simulink model "canBusModel"  (R2024b)
settings: Solver=FixedStepDiscrete  StartTime=0.0  StopTime=2  FixedStep=0.00001  RelTol=1e-3
undefined symbols (not defined in the file): CanFDSpeed_bps, CanSpeed_bps, FixedStep_us
settings Model: Creator=junho  LastModifiedBy=hrkim
settings DebuggingCC: ModelReferenceSymbolNameMessage=none
settings HardwareCC: TargetBitPerLong=64  TargetBitPerPointer=64  TargetBitPerSizeT=64  TargetBitPerPtrDiffT=64  TargetLongLongMode=on  TargetIntDivRoundTo=Zero  TargetEndianess=LittleEndian  TargetWordSize=64  TargetHWDeviceType=MATLAB Host  ProdEqTarget=off
settings SFSimCC: SimUserSources=../src/canBus.c  DefaultCustomCodeDeterministicFunctions=ByFunction  CustomCodeDeterministicFunctions=fmu_can_init
settings SFSimCC: SimCustomHeaderCode=|
  | #include "../src/canBus.h";
  | #include "string.h";
settings RTWCC: Description=FMU2CS  SystemTargetFile=fmu2cs.tlc  TemplateMakefile=fmu2cs_default_tmf  RTWVerbose=off  RTWUseSimCustomCode=on  CustomSource=../src/canBus.c  GPUComputeCapability=3.5
settings RTWCC: CustomHeaderCode=|
  | #include "../src/canBus.h";
  | #include "string.h";
settings CodeAppCC: MaxIdLength=255
settings GRTTargetCC: MatFileLogging=off

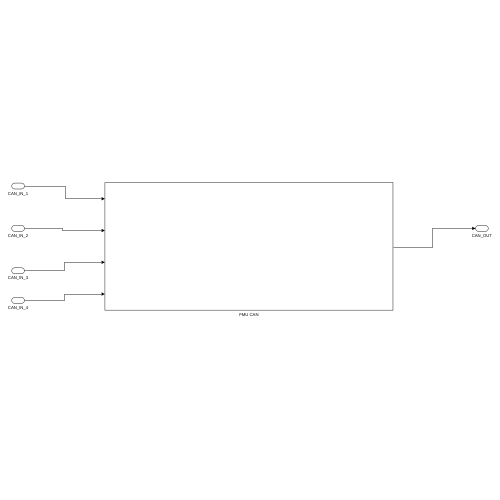
[thumbnail: Simulink's stored preview of the top-level diagram]
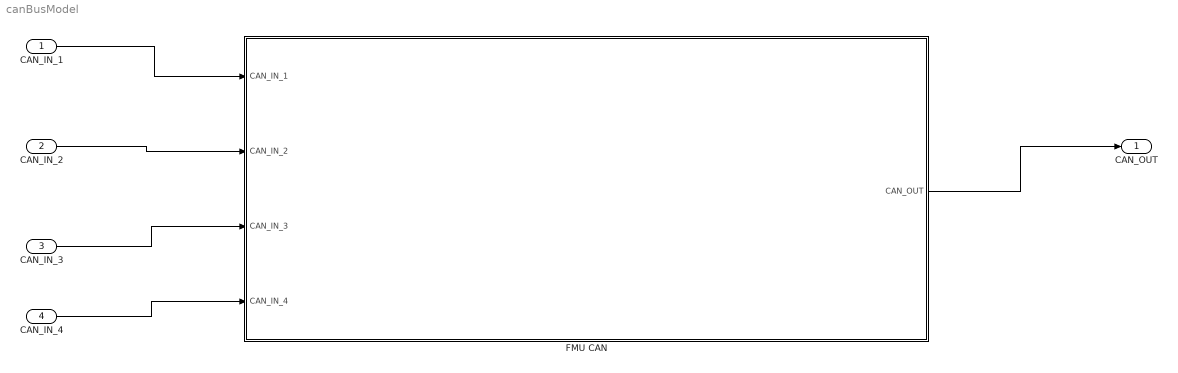
== system canBusModel ==
  CAN_IN_1 : Inport
  CAN_IN_2 : Inport  Port=2
  CAN_IN_3 : Inport  Port=3
  CAN_IN_4 : Inport  Port=4
  FMU CAN : Subsystem
  CAN_OUT : Outport
  wires:
  FMU CAN/1(CAN_OUT) -> CAN_OUT/1
  CAN_IN_1/1 -> FMU CAN/1(CAN_IN_1)
  CAN_IN_2/1 -> FMU CAN/2(CAN_IN_2)
  CAN_IN_3/1 -> FMU CAN/3(CAN_IN_3)
  CAN_IN_4/1 -> FMU CAN/4(CAN_IN_4)

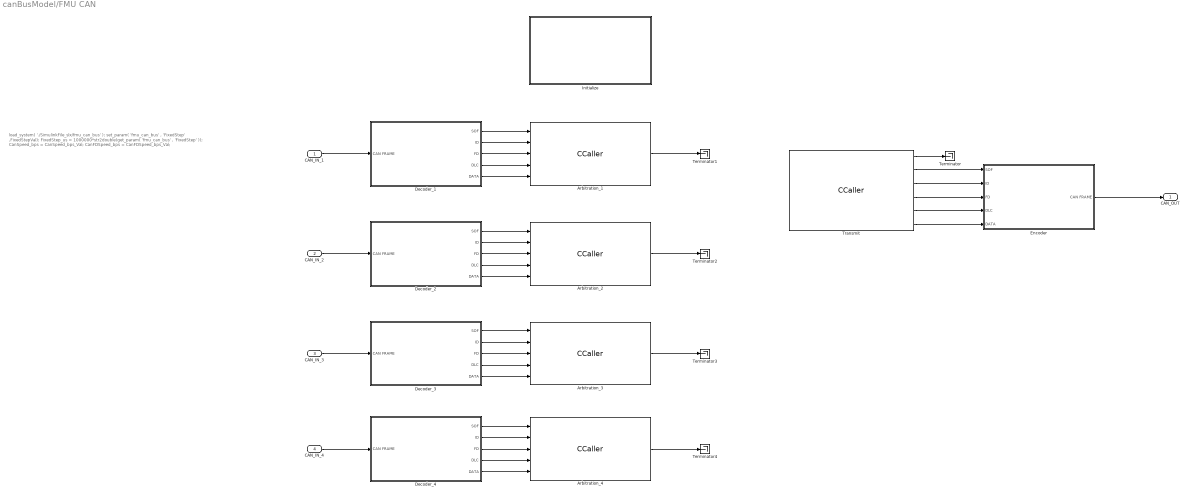
== system canBusModel/FMU CAN ==
  note: load_system( './SimulinkFile_slx/fmu_can_bus' );
      | set_param( 'fmu_can_bus' , 'FixedStep' ,FixedStepVal);
      | FixedStep_us = 1000000*str2double(get_param( 'fmu_can_bus' , 'FixedStep' ));
      | CanSpeed_bps = CanSpeed_bps_Val;
      | CanFDSpeed_bps = CanFDSpeed_bps_Val;
  CAN_IN_1 : Inport
  CAN_IN_2 : Inport  Port=2
  CAN_IN_3 : Inport  Port=3
  CAN_IN_4 : Inport  Port=4
  Arbitration_{1..4} (4 alike) : CCaller  Priority=1  FunctionName=fmu_can_arbitration  PortSpecificationStruct="%)30     .    . H   8    (     @         %    \"     8    !     0         %  0 \"0    $    _    07)G3F%M90  4&]R=$YA;64 4V-O<&4     26YD97@     5'EP90      4VEZ90      27-';&]B86P   X    P    !@    @    $          4    (     0    ,    !         !   P!O=70 #@   #     &    \"     0         !0    @    !     P    $         $  # &]U=  .    .     8    (    !          %    \"     $    &     0         0   ...(+3147 chars)"
  Decoder_1 : Subsystem
  Decoder_2 : Subsystem
  Decoder_3 : Subsystem
  Decoder_4 : Subsystem
  Encoder : Subsystem
  Initialize : Subsystem  TreatAsAtomicUnit=on
  Terminator{,1..4} (5 alike) : Terminator
  Transmit : CCaller  Priority=2  FunctionName=fmu_can_transmit  PortSpecificationStruct="%)30     .    . H   8    (     @         %    \"     8    !     0         %  0 \"0    $    _    07)G3F%M90  4&]R=$YA;64 4V-O<&4     26YD97@     5'EP90      4VEZ90      27-';&]B86P   X    P    !@    @    $          4    (     0    ,    !         !   P!O=70 #@   #     &    \"     0         !0    @    !     P    $         $  # &]U=  .    .     8    (    !          %    \"     $    &     0         0   ...(+3143 chars)"
  CAN_OUT : Outport
  wires:
  Arbitration_1/1 -> Terminator1/1
  Arbitration_2/1 -> Terminator2/1
  Transmit/1 -> Terminator/1
  CAN_IN_1/1 -> Decoder_1/1(CAN FRAME)
  CAN_IN_2/1 -> Decoder_2/1(CAN FRAME)
  Encoder/1(CAN FRAME) -> CAN_OUT/1
  Decoder_1/1(SOF) -> Arbitration_1/1
  Decoder_1/2(ID) -> Arbitration_1/2
  Decoder_1/3(FD) -> Arbitration_1/3
  Decoder_1/4(DLC) -> Arbitration_1/4
  Decoder_1/5(DATA) -> Arbitration_1/5
  Decoder_2/1(SOF) -> Arbitration_2/1
  Decoder_2/2(ID) -> Arbitration_2/2
  Decoder_2/3(FD) -> Arbitration_2/3
  Decoder_2/4(DLC) -> Arbitration_2/4
  Decoder_2/5(DATA) -> Arbitration_2/5
  Transmit/2 -> Encoder/1(SOF)
  Transmit/3 -> Encoder/2(ID)
  Transmit/4 -> Encoder/3(FD)
  Transmit/5 -> Encoder/4(DLC)
  Transmit/6 -> Encoder/5(DATA)
  CAN_IN_3/1 -> Decoder_3/1(CAN FRAME)
  Decoder_3/1(SOF) -> Arbitration_3/1
  Decoder_3/4(DLC) -> Arbitration_3/4
  Decoder_3/5(DATA) -> Arbitration_3/5
  Decoder_3/2(ID) -> Arbitration_3/2
  Arbitration_3/1 -> Terminator3/1
  Decoder_3/3(FD) -> Arbitration_3/3
  Decoder_4/2(ID) -> Arbitration_4/2
  Decoder_4/5(DATA) -> Arbitration_4/5
  Decoder_4/4(DLC) -> Arbitration_4/4
  Arbitration_4/1 -> Terminator4/1
  Decoder_4/3(FD) -> Arbitration_4/3
  CAN_IN_4/1 -> Decoder_4/1(CAN FRAME)
  Decoder_4/1(SOF) -> Arbitration_4/1

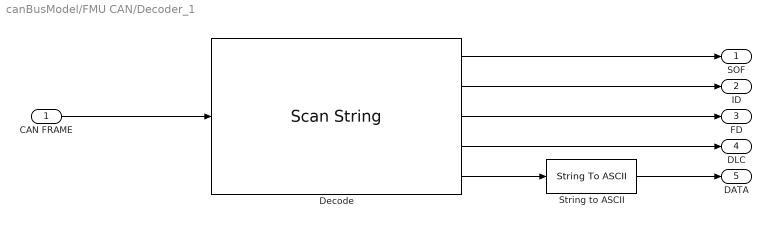
== system canBusModel/FMU CAN/Decoder_1 ==
  CAN FRAME : Inport
  Decode : ScanString  Format="\"%d-%d-%d-%d-%s\""
  String to ASCII : StringToASCII  OutputVectorSize=200
  SOF : Outport
  ID : Outport  Port=2
  FD : Outport  Port=3
  DLC : Outport  Port=4
  DATA : Outport  Port=5
  wires:
  CAN FRAME/1 -> Decode/1
  Decode/1 -> SOF/1
  Decode/2 -> ID/1
  Decode/3 -> FD/1
  Decode/5 -> String to ASCII/1
  String to ASCII/1 -> DATA/1
  Decode/4 -> DLC/1

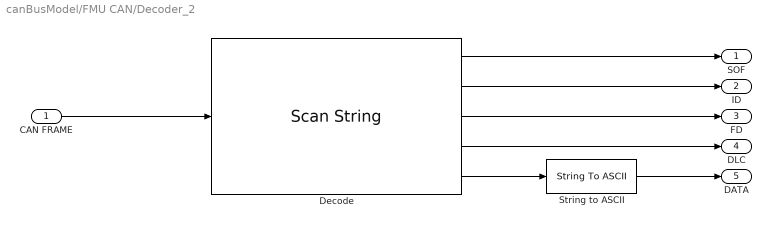
== system canBusModel/FMU CAN/Decoder_2 ==
  CAN FRAME : Inport
  Decode : ScanString  Format="\"%d-%d-%d-%d-%s\""
  String to ASCII : StringToASCII  OutputVectorSize=200
  SOF : Outport
  ID : Outport  Port=2
  FD : Outport  Port=3
  DLC : Outport  Port=4
  DATA : Outport  Port=5
  wires:
  Decode/4 -> DLC/1
  String to ASCII/1 -> DATA/1
  Decode/5 -> String to ASCII/1
  Decode/3 -> FD/1
  Decode/2 -> ID/1
  Decode/1 -> SOF/1
  CAN FRAME/1 -> Decode/1

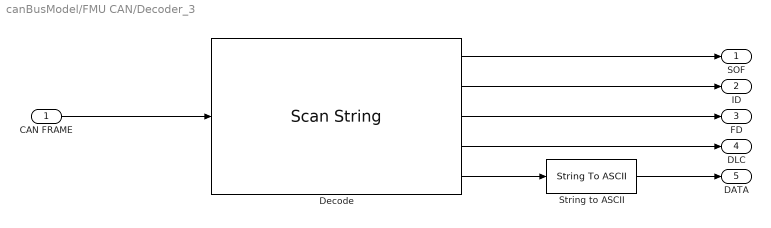
== system canBusModel/FMU CAN/Decoder_3 ==
  CAN FRAME : Inport
  Decode : ScanString  Format="\"%d-%d-%d-%d-%s\""
  String to ASCII : StringToASCII  OutputVectorSize=200
  SOF : Outport
  ID : Outport  Port=2
  FD : Outport  Port=3
  DLC : Outport  Port=4
  DATA : Outport  Port=5
  wires:
  Decode/4 -> DLC/1
  String to ASCII/1 -> DATA/1
  Decode/5 -> String to ASCII/1
  Decode/3 -> FD/1
  Decode/2 -> ID/1
  Decode/1 -> SOF/1
  CAN FRAME/1 -> Decode/1

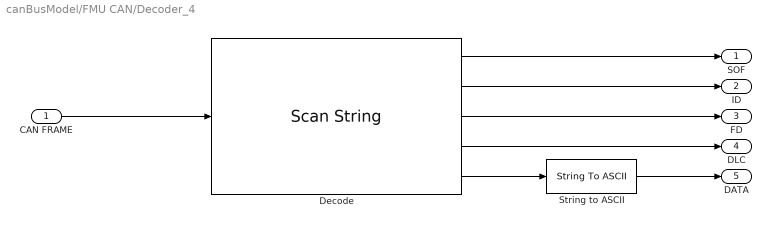
== system canBusModel/FMU CAN/Decoder_4 ==
  CAN FRAME : Inport
  Decode : ScanString  Format="\"%d-%d-%d-%d-%s\""
  String to ASCII : StringToASCII  OutputVectorSize=200
  SOF : Outport
  ID : Outport  Port=2
  FD : Outport  Port=3
  DLC : Outport  Port=4
  DATA : Outport  Port=5
  wires:
  Decode/4 -> DLC/1
  String to ASCII/1 -> DATA/1
  Decode/5 -> String to ASCII/1
  Decode/3 -> FD/1
  Decode/2 -> ID/1
  Decode/1 -> SOF/1
  CAN FRAME/1 -> Decode/1

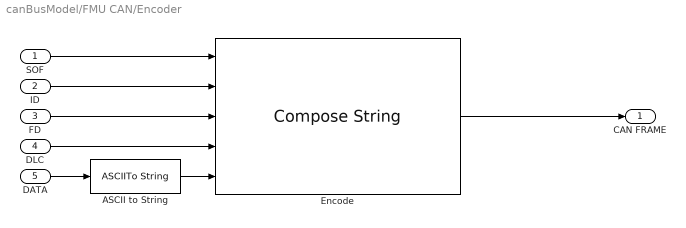
== system canBusModel/FMU CAN/Encoder ==
  SOF : Inport
  ID : Inport  Port=2
  FD : Inport  Port=3
  DLC : Inport  Port=4
  DATA : Inport  Port=5
  ASCII to String : ASCIIToString
  Encode : ComposeString  Format="\"%d-%d-%d-%d-%s\""
  CAN FRAME : Outport
  wires:
  SOF/1 -> Encode/1
  ID/1 -> Encode/2
  FD/1 -> Encode/3
  Encode/1 -> CAN FRAME/1
  DATA/1 -> ASCII to String/1
  ASCII to String/1 -> Encode/5
  DLC/1 -> Encode/4

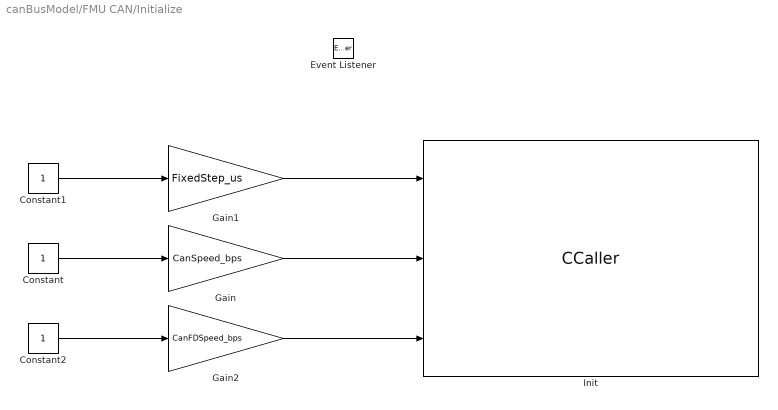
== system canBusModel/FMU CAN/Initialize ==
  Constant : Constant  OutDataTypeStr=int32
  Constant1 : Constant  OutDataTypeStr=int32
  Constant2 : Constant  OutDataTypeStr=int32
  Event Listener : EventListener  DisableCoverage=on  EventName=reset
  Gain : Gain  Gain=CanSpeed_bps  ParamDataTypeStr=int32  OutDataTypeStr=int32
  Gain1 : Gain  Gain=FixedStep_us  ParamDataTypeStr=int32  OutDataTypeStr=int32
  Gain2 : Gain  Gain=CanFDSpeed_bps  ParamDataTypeStr=int32  OutDataTypeStr=int32
  Init : CCaller  FunctionName=fmu_can_init  PortSpecificationStruct="%)30     .    N 4   8    (     @         %    \"     ,    !     0         %  0 \"0    $    _    07)G3F%M90  4&]R=$YA;64 4V-O<&4     26YD97@     5'EP90      4VEZ90      27-';&]B86P   X   !     !@    @    $          4    (     0    P    !         !     ,    9FEX961S=&5P7W5S      X   !     !@    @    $          4    (     0    P    !         !     ,    9FEX961S=&5P7W5S      X    X    !@    @    $          4    (     0    4    !         !     %    26YP=70    .    .     8    (    !@         %    \"     $    !     0         )    \"               #@   #@    &    \"     0         !0    @    !    !0    $         $     4   !I;G0S,@    X    P    !@    @    $          4    (     0    $    !         !   0 Q    #@   #     &    \"     D\"        !0    @    !     0    $          @ !       .    0     8    (    !          %    \"     $    -     0         0    #0   &-A;E]S<&5E9%]B<',    .    0     8    (    !          %    \"     $    -     0         0    #0   &-A;E]S<&5E9%]B<',    .    .     8    (    !          %    \"     $    %     0         0    !0   $EN<'5T    #@   #@    &    \"     8         !0    @    !     0    $         \"0    @           #P/PX    X    !@    @    $          4    (     0    4    !         !     %    :6YT,S(    .    ,     8    (    !          %    \"     $    !     0         0  $ ,0    X    P    !@    @    ) @        4    (     0    $    !          (  0      #@   $     &    \"     0         !0    @    !    #P    $         $     \\   !C86YF9%]S<&5E9%]B<', #@   $     &    \"     0         !0    @    !    #P    $         $     \\   !C86YF9%]S<&5E9%]B<', #@   #@    &    \"     0         !0    @    !    !0    $         $     4   !);G!U=     X    X    !@    @    &          4    (     0    $    !          D    (             $ .    .     8    (    !          %    \"     $    %     0         0    !0   &EN=#,R    #@   #     &    \"     0         !0    @    !     0    $         $  ! #$    .    ,     8    (    \"0(        %    \"     $    !     0         \"  $"
  wires:
  Constant/1 -> Gain/1
  Constant1/1 -> Gain1/1
  Gain1/1 -> Init/1
  Gain/1 -> Init/2
  Constant2/1 -> Gain2/1
  Gain2/1 -> Init/3
